simulink model "anfis_drone_sim2"  (R2024b)
settings: Solver=VariableStepAuto  StartTime=0.0  StopTime=10.0  RelTol=1e-3
values from neighbouring files (symbols this model uses):
  obstacles = [5 5 0.5 ... (first row only)    [dataset_cre2.m]
undefined symbols (not defined in the file or in its folder): endPoint, minVal, rangeVal, v_nom
libraries: fuzblock x1
settings Model: Creator=shuha  LastModifiedBy=shuha
settings ConfigComp: CovBoundaryAbsTol=1.0e-5

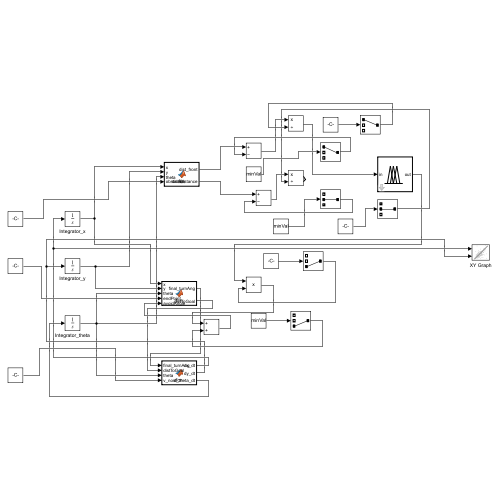
[thumbnail: Simulink's stored preview of the top-level diagram]
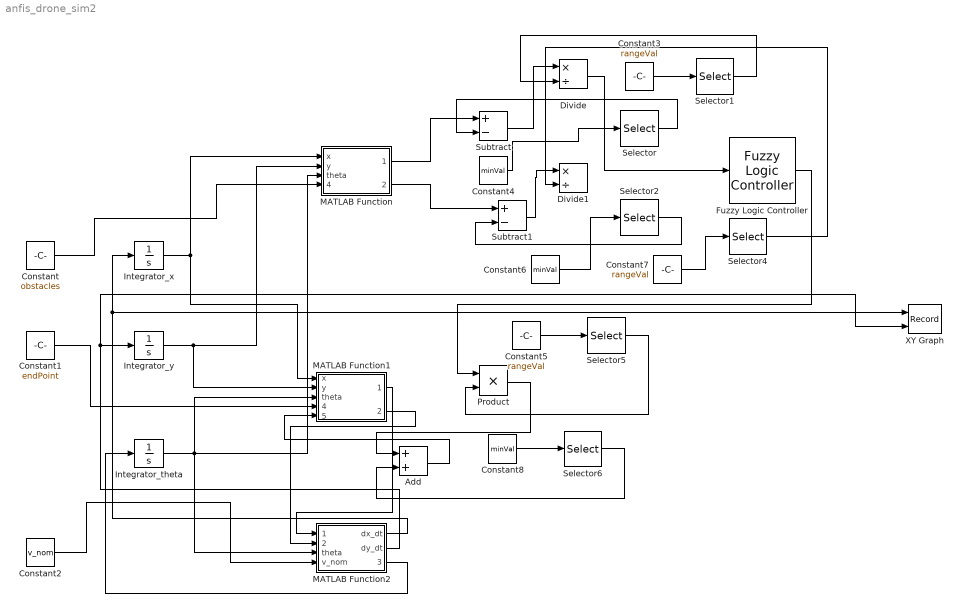
== system anfis_drone_sim2 ==
  Add : Sum
  Constant : Constant  Value=obstacles
  Constant1 : Constant  Value=endPoint
  Constant2 : Constant  Value=v_nom
  Constant3 : Constant  Value=rangeVal
  Constant4 : Constant  Value=minVal
  Constant5 : Constant  Value=rangeVal
  Constant6 : Constant  Value=minVal
  Constant7 : Constant  Value=rangeVal
  Constant8 : Constant  Value=minVal
  Divide : Product  Inputs=*/
  Divide1 : Product  Inputs=*/
  Fuzzy Logic Controller : fuzblock/Fuzzy Logic  Controller  FIS='traineddroneanfis.fis'  OutputSampleNumber=101  DataType=double  FuzzifiedInputs=off  RuleFiringStrengths=off  RuleOutputs=off  AggregatedOutputs=off  SimulateUsing=Interpreted execution  OutOfRangeInputValueMessage=warning  NoRuleFiredMessage=warning  EmptyOutputFuzzySetMessage=warning
  Integrator_theta : Integrator
  Integrator_x : Integrator  InitialCondition=-12
  Integrator_y : Integrator
  MATLAB Function : MATLAB Function  TreatAsAtomicUnit=on
  MATLAB Function1 : MATLAB Function  TreatAsAtomicUnit=on
  MATLAB Function2 : MATLAB Function  TreatAsAtomicUnit=on
  Product : Product
  Selector : Selector  InputPortWidth=3  IndexOptions=Index vector (dialog)  Indices=[1]  OutputSizes=1
  Selector1 : Selector  InputPortWidth=3  IndexOptions=Index vector (dialog)  Indices=[1]  OutputSizes=1
  Selector2 : Selector  InputPortWidth=3  IndexOptions=Index vector (dialog)  Indices=[2]  OutputSizes=1
  Selector4 : Selector  InputPortWidth=3  IndexOptions=Index vector (dialog)  Indices=[2]  OutputSizes=1
  Selector5 : Selector  InputPortWidth=3  IndexOptions=Index vector (dialog)  Indices=[3]  OutputSizes=1
  Selector6 : Selector  InputPortWidth=3  IndexOptions=Index vector (dialog)  Indices=[3]  OutputSizes=1
  Subtract : Sum  Inputs=+-
  Subtract1 : Sum  Inputs=+-
  XY Graph : Record  FileSettingsInternal="{\"entries\":[{\"content\":{\"excelSettings\":{\"content\":{},\"type\":\"Streamout.ExcelSettings\"},\"parquetSettings\":{\"content\":{},\"type\":\"Streamout.ParquetSettings\"}},\"type\":\"Streamout.FileSettingStorage\",\"uuid\":\"\"}],\"packageUris\":[\"http:\\/\\/schema.mathworks.com\\/mf0\\/streamout_blocks\\/R2020a\"],\"version\":\"1.0\"}"  Layout=[1 1]  SignalsInternal="{\"entries\":[{\"content\":{\"signals\":[{\"content\":{\"blockPath\":[],\"dimensions\":[1],\"domain\":\"\",\"lineColor\":\"#a2142f\",\"plots\":[ 1 ],\"port\":1,\"signalID\":1,\"signalName\":\"XY Graph:1\"},\"type\":\"RecordBlkView.Signal\",\"uuid\":\"\"},{\"content\":{\"blockPath\":[],\"dimensions\":[1],\"domain\":\"\",\"lineColor\":\"#139fff\",\"plots\":[ 1 ],\"port\":2,\"signalID\":2,\"signalName\":\"XY Graph:2\"},\"type\":\"RecordBlkView.Signal\",\"uuid\":\"\"}]},\"type\":\"RecordBlkView.InputSignals\",\"uuid\":\"\"}],\"packageUris\":[\"http:\\/\\/schema.mathworks.com\\/mf0\\/streamout_blocks\\/R2020a\"],\"version\":\"1.0\"}"  VisualizationBindings="{\"xyplotplugin\":{\"info\":[{\"series\":[{\"bindingParametersList\":[{\"parameter\":\"X-Axis\",\"signalID\":1,\"signalName\":\"XY Graph:1\"},{\"parameter\":\"Y-Axis\",\"signalID\":2,\"signalName\":\"XY Graph:2\"}],\"seriesID\":0}],\"subplotID\":1}]}}"  CompatibilityTag=XY
  wires:
  Integrator_x/1 -> MATLAB Function1/1(x), MATLAB Function/1(x)
  Integrator_y/1 -> MATLAB Function1/2(y), MATLAB Function/2(y)
  Integrator_theta/1 -> MATLAB Function2/3(theta), MATLAB Function1/3(theta), MATLAB Function/3(theta)
  Constant/1 -> MATLAB Function/4(obstacles)
  Constant1/1 -> MATLAB Function1/4(endPoint)
  Constant2/1 -> MATLAB Function2/4(v_nom)
  MATLAB Function/1(dist_front) -> Subtract/1
  Constant4/1 -> Selector/1
  Selector/1 -> Subtract/2
  Subtract/1 -> Divide/1
  Constant3/1 -> Selector1/1
  Selector1/1 -> Divide/2
  MATLAB Function/2(sideDistance) -> Subtract1/1
  Selector2/1 -> Subtract1/2
  Subtract1/1 -> Divide1/1
  Constant6/1 -> Selector2/1
  Constant7/1 -> Selector4/1
  Selector4/1 -> Divide1/2
  Fuzzy Logic Controller/1 -> Product/1
  Product/1 -> Add/1
  Constant5/1 -> Selector5/1
  Add/1 -> MATLAB Function1/5(avoidAngle)
  Selector5/1 -> Product/2
  Constant8/1 -> Selector6/1
  Selector6/1 -> Add/2
  MATLAB Function1/1(final_turnAng) -> MATLAB Function2/1(final_turnAng)
  MATLAB Function1/2(distToGoal) -> MATLAB Function2/2(distToGoal)
  MATLAB Function2/1(dx_dt) -> Integrator_x/1, XY Graph/1
  MATLAB Function2/2(dy_dt) -> XY Graph/2, Integrator_y/1
  MATLAB Function2/3(d_theta_dt) -> Integrator_theta/1
  Divide/1 -> Fuzzy Logic Controller/1

== matlab function anfis_drone_sim2/MATLAB Function1 ==
  data: x input; final_turnAng output; y input; theta input; endPoint input; avoidAngle input; distToGoal output
function [final_turnAng, distToGoal] = fcn(x, y, theta, endPoint, avoidAngle)
    % --- This code is from your script's Section 6 ---
    w_goal_base = 0.4;
    w_avoid_base = 0.6;
    goal_influence_radius = 5.0;

    distToGoal = sqrt((x - endPoint(1))^2 + (y - endPoint(2))^2);
    angleToGoal = rad2deg(atan2(endPoint(2) - y, endPoint(1) - x));
    goalSteer = mod(angleToGoal - rad2deg(theta) + 180, 360) - 180;

    if distToGoal < goal_influence_radius
        w_goal = 1.0 - (distToGoal / goal_influence_radius) * (1 - w_goal_base);
        w_avoid = 1.0 - w_goal;
    else
        w_goal = w_goal_base;
        w_avoid = w_avoid_base;
    end
    final_turnAng = w_goal * goalSteer + w_avoid * avoidAngle;

== matlab function anfis_drone_sim2/MATLAB Function ==
  data: x input; dist_front output; y input; theta input; obstacles input; sideDistance output
function [dist_front, sideDistance] = fcn(x, y, theta, obstacles)
    % --- This code is from your script's Section 6 ---
    dx = obstacles(:,1) - x;
    dy = obstacles(:,2) - y;
    dists = sqrt(dx.^2 + dy.^2);
    bearings = rad2deg(atan2(dy,dx)) - rad2deg(theta);
    bearings = mod(bearings + 180, 360) - 180;

    frontIdx = abs(bearings) <= 30;
    leftIdx = (bearings > 30) & (bearings <= 150);
    rightIdx = (bearings < -30) & (bearings >= -150);

    if any(frontIdx), dist_front = min(dists(frontIdx)); else, dist_front = 20; end
    if any(leftIdx), dist_left = min(dists(leftIdx)); else, dist_left = 20; end
    if any(rightIdx), dist_right = min(dists(rightIdx)); else, dist_right = 20; end

    sideDistance = min(dist_left, dist_right);

== matlab function anfis_drone_sim2/MATLAB Function2 ==
  data: final_turnAng input; dx_dt output; distToGoal input; theta input; v_nom input; dy_dt output; d_theta_dt output
function [dx_dt, dy_dt, d_theta_dt] = fcn(final_turnAng, distToGoal, theta, v_nom)
    % --- This code is from your script's Section 6 ---
    v = min(v_nom, distToGoal);
    v = max(v, 0.1);

    % This is d(theta)/dt
    yawRateRad = deg2rad(max(min(final_turnAng, 60), -60));
    d_theta_dt = yawRateRad; 

    % This is dx/dt
    dx_dt = v * cos(theta);  

    % This is dy/dt
    dy_dt = v * sin(theta);
